simulink model "motormodel"  (Simulink 10.2)
settings: Solver=ode45  StartTime=0.0  StopTime=8  RelTol=1e-3  EnableMultiTasking=on
PreLoadFcn:
  | MotorParam
InitFcn:
  | MotorParam
values from neighbouring files (symbols this model uses):
  B = Km * 0.0392 / 649.262481742    (= 5.54253495496e-07)    [MotorParam.m]    (also in TFandRL.m)
  J = 0.000000505 + 0.000012203355624    (= 1.2708355624e-05)    [MotorParam.m]    (also in TFandRL.m)
  Kb = 0.00918    [MotorParam.m]    (also in TFandRL.m)
  Km = 0.00918    [MotorParam.m]    (also in TFandRL.m)
  L = 0.000058    (= 5.8e-05)    [MotorParam.m]    (also in TFandRL.m)
  R = 1.02    [MotorParam.m]    (also in TFandRL.m)
settings Model: Creator=Leo  LastModifiedBy=tnurs
settings DataIOCC: LimitDataPoints=on
settings OptimizationCC: ExpressionDepthLimit=2147483647  InitFltsAndDblsToZero=on
settings DebuggingCC: SolverPrmCheckMsg=warning  StateNameClashWarn=warning
settings ConfigComp: CovSFcnEnable=off

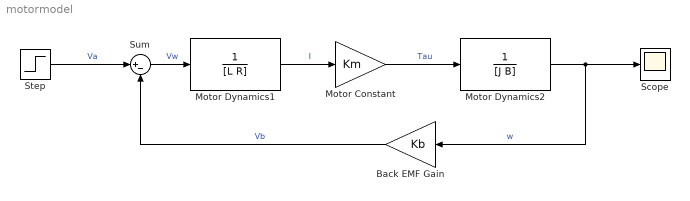
== system motormodel ==
  Back EMF Gain : Gain  Gain=Kb
  Motor Constant : Gain  Gain=Km
  Motor Dynamics1 : TransferFcn  Denominator=[L R]
  Motor Dynamics2 : TransferFcn  Denominator=[J B]
  Scope : Scope
  Step : Step  After=6  SampleTime=0
  Sum : Sum  Inputs=|+-
  wires:
  Step/1 -> Sum/1  "Va"
  Sum/1 -> Motor Dynamics1/1  "Vw"
  Motor Dynamics1/1 -> Motor Constant/1  "I"
  Motor Constant/1 -> Motor Dynamics2/1  "Tau"
  Motor Dynamics2/1 -> Scope/1, Back EMF Gain/1  "w"
  Back EMF Gain/1 -> Sum/2  "Vb"
